simulink model "shunt_a"  (R2019a)
settings: Solver=VariableStepAuto  StartTime=0.0  StopTime=10.0  RelTol=1e-3
undefined symbols (not defined in the file): Bm, LAF, ra, rf, Tl, Va
libraries: fl_lib x15, nesl_utility x10
settings Model: Creator=azizi  LastModifiedBy=azizi

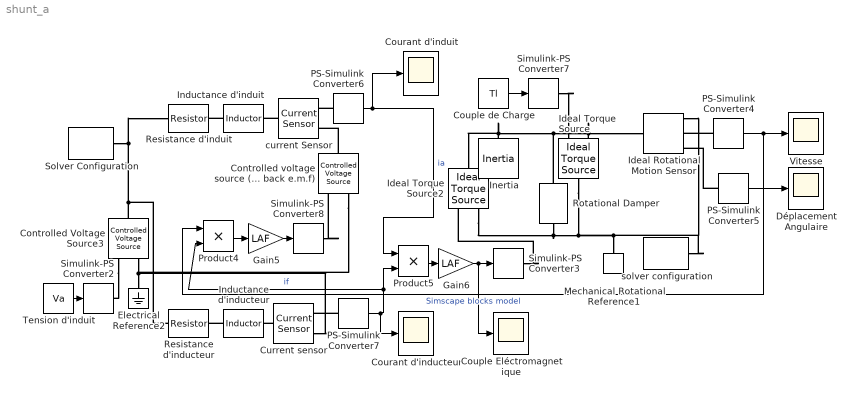
== system shunt_a ==
  " Ideal Torque Source" : fl_lib/Mechanical/Mechanical Sources/Ideal Torque Source
  Controlled voltage source (i.e. back e.m.f) : fl_lib/Electrical/Electrical Sources/Controlled Voltage Source
  Controlled Voltage Source3 : fl_lib/Electrical/Electrical Sources/Controlled Voltage Source
  Couple Eléctromagnetique : Scope
  Couple de Charge : Constant  Value=Tl
  Courant d'inducteur : Scope
  Courant d'induit : Scope
  Current sensor : fl_lib/Electrical/Electrical Sensors/Current Sensor
  Déplacement Angulaire : Scope
  Electrical Reference2 : fl_lib/Electrical/Electrical Elements/Electrical Reference
  Gain5 : Gain  Gain=LAF
  Gain6 : Gain  Gain=LAF
  Ideal Rotational Motion Sensor : fl_lib/Mechanical/Mechanical Sensors/Ideal Rotational Motion Sensor  offset=0 rev
  Ideal Torque Source2 : fl_lib/Mechanical/Mechanical Sources/Ideal Torque Source
  Inductance d'inducteur : fl_lib/Electrical/Electrical Elements/Inductor  l=LFF H  r=0 Ohm  g=0 1/Ohm  i_specify=off  i_priority=None  i=0 A  i_nominal_specify=off  i_nominal_unit=A  i_nominal_value=1  v_specify=off  v_priority=None  v=0 V  v_nominal_specify=off  v_nominal_unit=V  v_nominal_value=1  i_L_specify=off  i_L_priority=High  i_L=0 A  i_L_nominal_specify=off  i_L_nominal_unit=A  i_L_nominal_value=1
  Inductance d'induit : fl_lib/Electrical/Electrical Elements/Inductor  l=LAA H  r=0 Ohm  g=0 1/Ohm  i_specify=off  i_priority=None  i=0 A  i_nominal_specify=off  i_nominal_unit=A  i_nominal_value=1  v_specify=off  v_priority=None  v=0 V  v_nominal_specify=off  v_nominal_unit=V  v_nominal_value=1  i_L_specify=off  i_L_priority=High  i_L=0 A  i_L_nominal_specify=off  i_L_nominal_unit=A  i_L_nominal_value=1
  "Inertia " : fl_lib/Mechanical/Rotational Elements/Inertia  inertia=J kg*m^2  w_specify=off  w_priority=High  w=0 rad/s  w_nominal_specify=off  w_nominal_unit=rad/s  w_nominal_value=1  t_specify=off  t_priority=None  t=0 N*m  t_nominal_specify=off  t_nominal_unit=N*m  t_nominal_value=1
  Mechanical Rotational Reference1 : fl_lib/Mechanical/Rotational Elements/Mechanical Rotational Reference
  PS-Simulink Converter{4..7} (4 alike) : nesl_utility/PS-Simulink Converter  PhysicalDomain=network_engine_domain  SubClassName=ps_output  LeftPortType=input  RightPortType=output  PseudoPeriodic=off  Frequencies=[]  Unit=1  AffineConversion=off
  Product4 : Product
  Product5 : Product
  Resistance d'inducteur : fl_lib/Electrical/Electrical Elements/Resistor  R=rf Ohm  i_specify=off  i_priority=None  i=0 A  i_nominal_specify=off  i_nominal_unit=A  i_nominal_value=1  v_specify=off  v_priority=None  v=0 V  v_nominal_specify=off  v_nominal_unit=V  v_nominal_value=1
  Resistance d'induit : fl_lib/Electrical/Electrical Elements/Resistor  R=ra Ohm  i_specify=off  i_priority=None  i=0 A  i_nominal_specify=off  i_nominal_unit=A  i_nominal_value=1  v_specify=off  v_priority=None  v=0 V  v_nominal_specify=off  v_nominal_unit=V  v_nominal_value=1
  "Rotational Damper  " : fl_lib/Mechanical/Rotational Elements/Rotational Damper  D=Bm N*m/(rad/s)  w_specify=off  w_priority=None  w=0 rad/s  w_nominal_specify=off  w_nominal_unit=rad/s  w_nominal_value=1  t_specify=off  t_priority=None  t=0 N*m  t_nominal_specify=off  t_nominal_unit=N*m  t_nominal_value=1
  Simulink-PS Converter{2..3,7..8} (4 alike) : nesl_utility/Simulink-PS Converter  PhysicalDomain=network_engine_domain  SubClassName=ps_input  LeftPortType=input  RightPortType=output  PseudoPeriodic=off  Frequencies=[]  NoiseDistribution=none  NoiseParameters=[]  Unit=1  AffineConversion=off  FilteringAndDerivatives=provide  SimscapeFilterOrder=1  InputFilterTimeConstant=0.001  UdotUserProvided=0
  Solver Configuration : nesl_utility/Solver Configuration  PhysicalDomain=network_engine_domain  SubClassName=solver  LeftPortType=input  RightPortType=generic  Tones=[]  Harmonics=[]  SimulateNoise=off  Profile=off  UseLocalSampling=off  EnableSwitchedLinearOptims=on  FrequencyDomain=off  UseCCode=off  RelTol=0.001  AbsTol=1e-06  MinStep=1e-09  ToWorkspace=off  RevertToSquareIcSolve=off  NumHomotopyIterations=100  PhasorMode=off  PhasorModeNumHarmonics=1  DoDC=off  ResidualTolerance=1e-09  UseLocalSolver=off  LocalSolverChoice=NE_BACKWARD_EULER_ADVANCER  LocalSolverSampleTime=0.001  DoFixedCost=off  MaxNonlinIter=3  MaxModeIter=2  LinearAlgebra=Sparse  EquationFormulation=NE_TIME_EF  DelaysMemoryBudget=1024  AutomaticFiltering=on  FilteringTimeConstant=0.001  PartitionStorageMethod=AS_NEEDED  PartitionMemoryBudget=1024  PartitionMethod=FAST
  Tension d'induit : Constant  Value=Va
  "Vitesse " : Scope
  "current Sensor " : fl_lib/Electrical/Electrical Sensors/Current Sensor
  solver configuration : nesl_utility/Solver Configuration  PhysicalDomain=network_engine_domain  SubClassName=solver  LeftPortType=input  RightPortType=generic  Tones=[]  Harmonics=[]  SimulateNoise=off  Profile=off  UseLocalSampling=off  EnableSwitchedLinearOptims=on  FrequencyDomain=off  UseCCode=off  RelTol=0.001  AbsTol=1e-06  MinStep=1e-09  ToWorkspace=off  RevertToSquareIcSolve=off  NumHomotopyIterations=100  PhasorMode=off  PhasorModeNumHarmonics=1  DoDC=off  ResidualTolerance=1e-09  UseLocalSolver=off  LocalSolverChoice=NE_BACKWARD_EULER_ADVANCER  LocalSolverSampleTime=0.001  DoFixedCost=off  MaxNonlinIter=3  MaxModeIter=2  LinearAlgebra=Sparse  EquationFormulation=NE_TIME_EF  DelaysMemoryBudget=1024  AutomaticFiltering=on  FilteringTimeConstant=0.001  PartitionStorageMethod=AS_NEEDED  PartitionMemoryBudget=1024  PartitionMethod=FAST
  wires:
  Couple de Charge/1 -> Simulink-PS Converter7/1
  PS-Simulink Converter7/1 -> Courant d'inducteur/1, Product5/2, Product4/2  "if"
  PS-Simulink Converter4/1 -> "Vitesse "/1, Product4/1  "Simscape blocks model"
  PS-Simulink Converter6/1 -> Courant d'induit/1, Product5/1  "ia"
  Gain5/1 -> Simulink-PS Converter8/1
  Tension d'induit/1 -> Simulink-PS Converter2/1
  Gain6/1 -> Couple Eléctromagnetique/1, Simulink-PS Converter3/1
  Product4/1 -> Gain5/1
  Product5/1 -> Gain6/1
  PS-Simulink Converter5/1 -> Déplacement Angulaire/1
  connections:
  Controlled Voltage Source3/LConn1 -- Resistance d'induit/LConn1 -- Solver Configuration/RConn1 -- Resistance d'inducteur/LConn1
  "Inertia "/LConn1 -- " Ideal Torque Source"/RConn2 -- Ideal Rotational Motion Sensor/LConn1 -- "Rotational Damper  "/LConn1 -- Ideal Torque Source2/LConn1
  Ideal Torque Source2/RConn2 -- " Ideal Torque Source"/LConn1 -- Ideal Rotational Motion Sensor/RConn1 -- solver configuration/RConn1 -- Mechanical Rotational Reference1/LConn1 -- "Rotational Damper  "/RConn1
  Electrical Reference2/LConn1 -- Controlled Voltage Source3/RConn2 -- Controlled voltage source (i.e. back e.m.f)/RConn2 -- Current sensor/RConn2
  Current sensor/LConn1 -- Inductance d'inducteur/RConn1
  PS-Simulink Converter4/LConn1 -- Ideal Rotational Motion Sensor/RConn2
  Inductance d'induit/LConn1 -- Resistance d'induit/RConn1
  PS-Simulink Converter5/LConn1 -- Ideal Rotational Motion Sensor/RConn3
  PS-Simulink Converter7/LConn1 -- Current sensor/RConn1
  PS-Simulink Converter6/LConn1 -- "current Sensor "/RConn1
  Controlled Voltage Source3/RConn1 -- Simulink-PS Converter2/RConn1
  Simulink-PS Converter3/RConn1 -- Ideal Torque Source2/RConn1
  "current Sensor "/LConn1 -- Inductance d'induit/RConn1
  Simulink-PS Converter7/RConn1 -- " Ideal Torque Source"/RConn1
  Inductance d'inducteur/LConn1 -- Resistance d'inducteur/RConn1
  Controlled voltage source (i.e. back e.m.f)/LConn1 -- "current Sensor "/RConn2
  Simulink-PS Converter8/RConn1 -- Controlled voltage source (i.e. back e.m.f)/RConn1
